simulink model "hil_vhf_model_setup"  (R2022b)
settings: Solver=FixedStepAuto  StartTime=0.0  StopTime=9  RelTol=1e-3
PreLoadFcn:
  | run('control_bus.m')
  | addpath('.\observers','.\control')
model workspace (MAT data in the model file):
  C = 39.8
  D = 0.05
  Lc = [1.1848250893; -624.760865246]
  M = 740
  Nd = 40
  Tmax = 1000
  a = 0.015
  esc_ic = 0.1
  g = 9.807
  h = 0.577
  l = 1.917
  lf = 1.036
  lr = 0.881
  omega = 100
  phi = -1.0471975512
  re = 0.284
  x0 = 200
  x_c = 90
  x_l = 10
undefined symbols (not defined in the file): Kalman, magnitude, r
libraries: simulink x2, Solver_SF x1
CloseFcn:
  | clear control_info_bus
settings Model: DataDictionary=kf_dict.sldd  Creator=henri  LastModifiedBy=Henrique Mesquita
settings DebuggingCC: UnconnectedInputMsg=warning  UnconnectedOutputMsg=warning  UnconnectedLineMsg=warning
settings ModelReferenceCC: EnableRefExpFcnMdlSchedulingChecks=on
settings SFSimCC: SimUserIncludeDirs="\".\\observers\""
settings RTWCC: DLArmComputeVersion=19.05

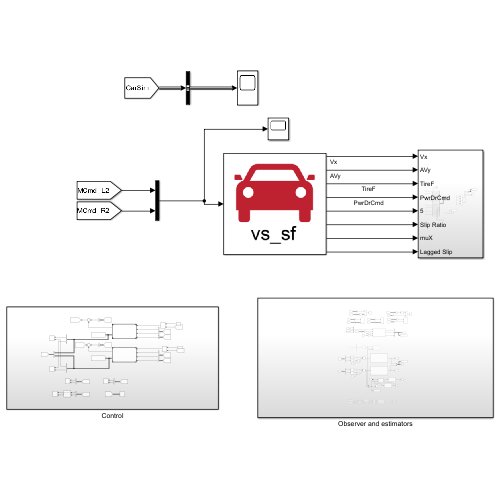
[thumbnail: Simulink's stored preview of the top-level diagram]
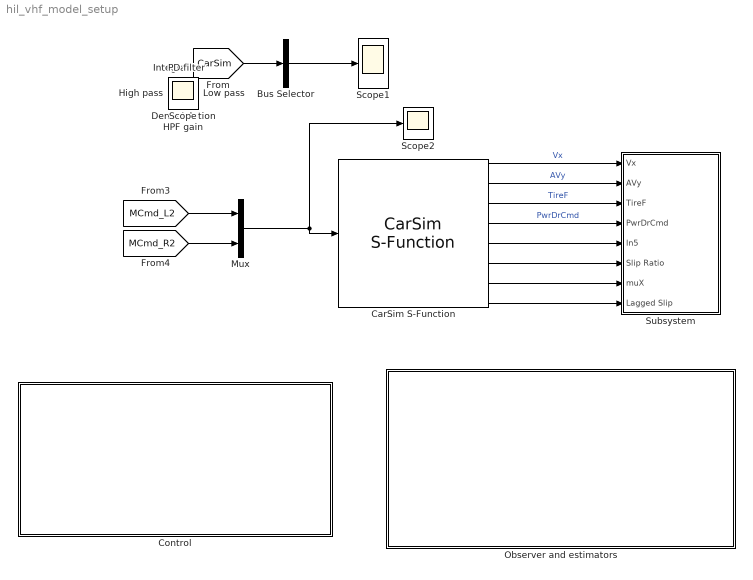
== system hil_vhf_model_setup ==
  Bus Selector : BusSelector  OutputSignals=AVy_L1,AVy_R1,AVy_L2,AVy_R2  OutputAsBus=on
  CarSim S-Function : Solver_SF/CarSim S-Function  Priority=1  SIMFILE=simfile.sim  Run_RTs=off  vs_state_ind=Run  StopMode_ind=Vehicle Model
  Control : Subsystem
  Mux : Mux  Inputs=2
  Observer and estimators : Subsystem
  Scope1 : Scope
  Scope2 : Scope
  Subsystem : Subsystem
  Demodulation : Scope
  HPF gain : Scope
  High pass : Scope
  Integrator : Scope
  Low pass : Scope
  PD filter : Scope
  Scope : Scope
  wires:
  Mux/1 -> Scope2/1, CarSim S-Function/1
  [CarSim] -> Bus Selector/1
  Bus Selector/1 -> Scope1/1
  CarSim S-Function/2 -> Subsystem/2(AVy)  "AVy"
  [MCmd_R2] -> Mux/2
  [MCmd_L2] -> Mux/1
  CarSim S-Function/6 -> Subsystem/6(Slip Ratio)
  CarSim S-Function/7 -> Subsystem/7(muX)
  CarSim S-Function/1 -> Subsystem/1(Vx)  "Vx"
  CarSim S-Function/3 -> Subsystem/3(TireF)  "TireF"
  CarSim S-Function/4 -> Subsystem/4(PwrDrCmd)  "PwrDrCmd"
  CarSim S-Function/5 -> Subsystem/5(In5)
  CarSim S-Function/8 -> Subsystem/8(Lagged Slip)

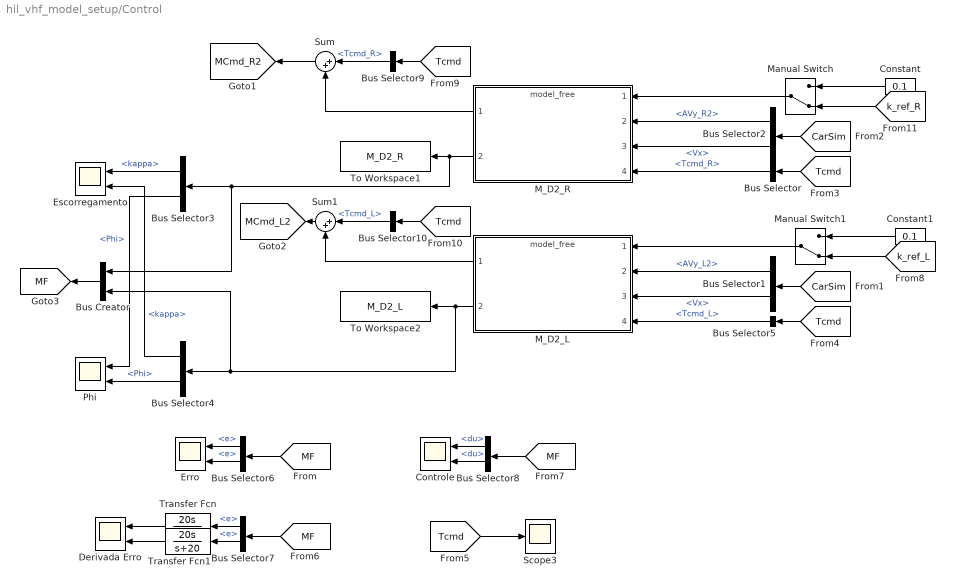
== system hil_vhf_model_setup/Control ==
  Bus Creator : BusCreator  Inputs=2
  Bus Selector : BusSelector  OutputSignals=Tcmd_R
  Bus Selector1 : BusSelector  OutputSignals=AVy_L2,Vx
  Bus Selector10 : BusSelector  OutputSignals=Tcmd_L
  Bus Selector2 : BusSelector  OutputSignals=AVy_R2,Vx
  Bus Selector3 : BusSelector  OutputSignals=kappa,Phi
  Bus Selector4 : BusSelector  OutputSignals=kappa,Phi
  Bus Selector5 : BusSelector  OutputSignals=Tcmd_L
  Bus Selector6 : BusSelector  OutputSignals=info (signal 1).e,info (signal 2).e
  Bus Selector7 : BusSelector  OutputSignals=info (signal 1).e,info (signal 2).e
  Bus Selector8 : BusSelector  OutputSignals=info (signal 1).du,info (signal 2).du
  Bus Selector9 : BusSelector  OutputSignals=Tcmd_R
  Constant : Constant  Value=0.1
  Constant1 : Constant  Value=0.1
  Controle : Scope  NumInputPorts=2
  Derivada Erro : Scope  NumInputPorts=2
  Erro : Scope  NumInputPorts=2
  "Escorregamento " : Scope  NumInputPorts=2
  M_D2_L : ModelReference  ModelNameDialog=model_free.slx  SimulationMode=Normal  ModelReferenceVersion=4.1
  M_D2_R : ModelReference  ModelNameDialog=model_free.slx  SimulationMode=Normal  ModelReferenceVersion=4.1
  Manual Switch : ManualSwitch  CurrentSetting=0
  Manual Switch1 : ManualSwitch  CurrentSetting=0
  Phi : Scope  NumInputPorts=2
  Scope3 : Scope
  Sum : Sum  Inputs=|++
  Sum1 : Sum  Inputs=|++
  To Workspace1 : ToWorkspace  VariableName=M_D2_R  SaveFormat=Timeseries  SampleTime=-1
  To Workspace2 : ToWorkspace  VariableName=M_D2_L  SaveFormat=Timeseries  SampleTime=-1
  Transfer Fcn : TransferFcn  Numerator=[20 0]  Denominator=[1 20]
  Transfer Fcn1 : TransferFcn  Numerator=[20 0]  Denominator=[1 20]
  tag scope: MCmd_L2=global, MCmd_R2=global, MF=global
  wires:
  M_D2_R/2 -> Bus Creator/1, Bus Selector3/1, To Workspace1/1
  Bus Selector3/1 -> "Escorregamento "/1  "<kappa>"
  Bus Selector1/1 -> M_D2_L/2  "<AVy_L2>"
  M_D2_L/2 -> Bus Creator/2, Bus Selector4/1, To Workspace2/1
  Manual Switch/1 -> M_D2_R/1
  Bus Selector4/2 -> Phi/2  "<Phi>"
  Bus Selector4/1 -> "Escorregamento "/2  "<kappa>"
  [CarSim] -> Bus Selector1/1
  Bus Selector3/2 -> Phi/1  "<Phi>"
  Bus Selector1/2 -> M_D2_L/3  "<Vx>"
  [CarSim] -> Bus Selector2/1
  Bus Selector2/1 -> M_D2_R/2  "<AVy_R2>"
  Bus Selector2/2 -> M_D2_R/3  "<Vx>"
  [Tcmd] -> Bus Selector/1
  Bus Selector/1 -> M_D2_R/4  "<Tcmd_R>"
  [Tcmd] -> Bus Selector5/1
  Bus Selector5/1 -> M_D2_L/4  "<Tcmd_L>"
  [Tcmd] -> Scope3/1
  [k_ref_R] -> Manual Switch/2
  Constant/1 -> Manual Switch/1
  Bus Creator/1 -> [MF]
  [MF] -> Bus Selector6/1
  Bus Selector6/1 -> Erro/1  "<e>"
  Bus Selector6/2 -> Erro/2  "<e>"
  [MF] -> Bus Selector7/1
  Bus Selector7/2 -> Transfer Fcn1/1  "<e>"
  Bus Selector7/1 -> Transfer Fcn/1  "<e>"
  Transfer Fcn/1 -> Derivada Erro/1
  Transfer Fcn1/1 -> Derivada Erro/2
  Bus Selector8/2 -> Controle/2  "<du>"
  Bus Selector8/1 -> Controle/1  "<du>"
  [MF] -> Bus Selector8/1
  Constant1/1 -> Manual Switch1/1
  [k_ref_L] -> Manual Switch1/2
  Manual Switch1/1 -> M_D2_L/1
  Sum/1 -> [MCmd_R2]
  [Tcmd] -> Bus Selector9/1
  Bus Selector9/1 -> Sum/1  "<Tcmd_R>"
  M_D2_R/1 -> Sum/2
  Bus Selector10/1 -> Sum1/1  "<Tcmd_L>"
  [Tcmd] -> Bus Selector10/1
  Sum1/1 -> [MCmd_L2]
  M_D2_L/1 -> Sum1/2

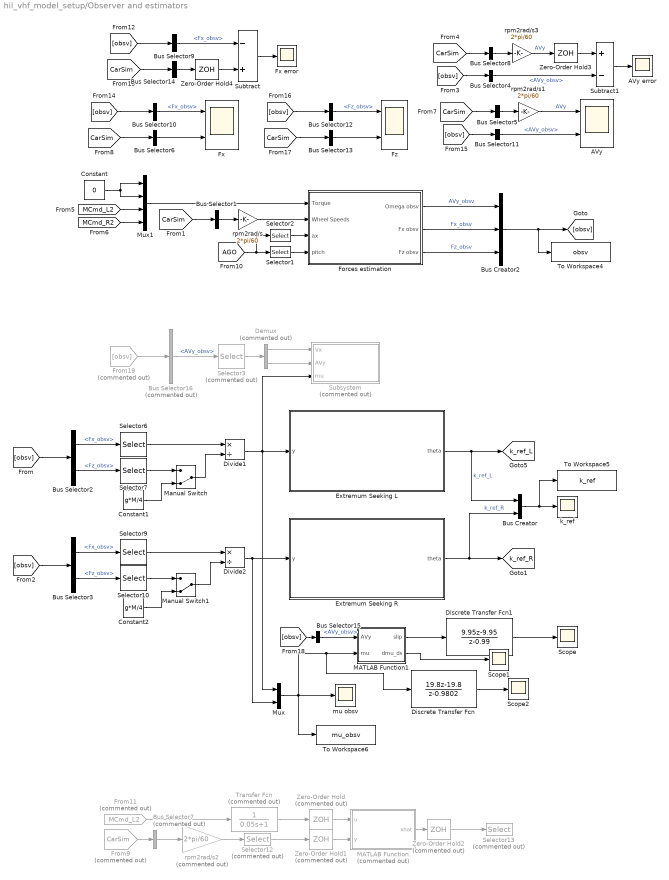
== system hil_vhf_model_setup/Observer and estimators ==
  AVy : Scope  NumInputPorts=2
  AVy error : Scope
  Bus Creator : BusCreator  Inputs=2
  Bus Creator2 : BusCreator  Inputs=3
  Bus Selector1 : BusSelector  OutputSignals=AVy_L1,AVy_R1,AVy_L2,AVy_R2  OutputAsBus=on
  Bus Selector10 : BusSelector  OutputSignals=Fx_obsv
  Bus Selector11 : BusSelector  OutputSignals=AVy_obsv
  Bus Selector12 : BusSelector  OutputSignals=Fz_obsv
  Bus Selector13 : BusSelector  OutputSignals=Fz_L1,Fz_R1,Fz_L2,Fz_R2  OutputAsBus=on
  Bus Selector14 : BusSelector  OutputSignals=Fx_L1,Fx_R1,Fx_L2,Fx_R2  OutputAsBus=on
  Bus Selector15 : BusSelector  OutputSignals=AVy_obsv
  Bus Selector16 : BusSelector  Commented=on  OutputSignals=AVy_obsv
  Bus Selector2 : BusSelector  OutputSignals=Fx_obsv,Fz_obsv
  Bus Selector3 : BusSelector  OutputSignals=Fx_obsv,Fz_obsv
  Bus Selector4 : BusSelector  OutputSignals=AVy_obsv
  Bus Selector5 : BusSelector  OutputSignals=AVy_L1,AVy_R1,AVy_L2,AVy_R2  OutputAsBus=on
  Bus Selector6 : BusSelector  OutputSignals=Fx_L1,Fx_R1,Fx_L2,Fx_R2  OutputAsBus=on
  Bus Selector7 : BusSelector  Commented=on  OutputSignals=AVy_L1,AVy_R1,AVy_L2,AVy_R2  OutputAsBus=on
  Bus Selector8 : BusSelector  OutputSignals=AVy_L1,AVy_R1,AVy_L2,AVy_R2  OutputAsBus=on
  Bus Selector9 : BusSelector  OutputSignals=Fx_obsv
  Constant : Constant  Value=0
  Constant1 : Constant  Value=g*M/4
  Constant2 : Constant  Value=g*M/4
  Demux : Demux  Commented=on  Outputs=2
  Discrete Transfer Fcn : DiscreteTransferFcn  Numerator=[19.8 -19.8]  Denominator=[1 -0.9802]
  Discrete Transfer Fcn1 : DiscreteTransferFcn  Numerator=[9.95 -9.95]  Denominator=[1 -0.99]
  Divide1 : Product  Inputs=*/
  Divide2 : Product  Inputs=*/
  Extremum Seeking L : Subsystem  Variant=on  VariantControlMode=label  VariantControl=Choice  LabelModeActiveChoice=ESC w/ vx gain  PropagateVariantConditions=on
  Extremum Seeking R : Subsystem  Variant=on  VariantControlMode=label  VariantControl=Choice  LabelModeActiveChoice=ESC w/ vx gain  PropagateVariantConditions=on
  Forces estimation : Subsystem  Variant=on  VariantControlMode=label  VariantControl=Choice  LabelModeActiveChoice=algebraic_PIO
  From11 : From  Commented=on  GotoTag=MCmd_L2  TagVisibility=global
  From19 : From  Commented=on  GotoTag=obsv
  From9 : From  Commented=on  GotoTag=CarSim  TagVisibility=global
  Fx : Scope  NumInputPorts=2
  Fx error : Scope
  Fz : Scope  NumInputPorts=2
  MATLAB Function : MATLAB Function  Commented=on  TreatAsAtomicUnit=on
  MATLAB Function1 : MATLAB Function  TreatAsAtomicUnit=on
  Manual Switch : ManualSwitch  CurrentSetting=0
  Manual Switch1 : ManualSwitch  CurrentSetting=0
  Mux : Mux  Inputs=2
  Mux1 : Mux
  Scope : Scope
  Scope1 : Scope
  Scope2 : Scope
  Selector1 : Selector  InputPortWidth=9  IndexOptions=Index vector (dialog)  Indices=[8]  OutputSizes=1
  Selector10 : Selector  InputPortWidth=4  IndexOptions=Index vector (dialog)  Indices=[4]  OutputSizes=1
  Selector12 : Selector  Commented=on  InputPortWidth=4  IndexOptions=Index vector (dialog)  Indices=[3]  OutputSizes=1
  Selector13 : Selector  Commented=on  InputPortWidth=2  IndexOptions=Index vector (dialog)  Indices=[2]  OutputSizes=1
  Selector2 : Selector  InputPortWidth=9  IndexOptions=Index vector (dialog)  Indices=[1]  OutputSizes=1
  Selector3 : Selector  Commented=on  InputPortWidth=4  IndexOptions=Index vector (dialog)  Indices=[1 3]  OutputSizes=1
  Selector6 : Selector  InputPortWidth=4  IndexOptions=Index vector (dialog)  Indices=[3]  OutputSizes=1
  Selector7 : Selector  InputPortWidth=4  IndexOptions=Index vector (dialog)  Indices=[3]  OutputSizes=1
  Selector9 : Selector  InputPortWidth=4  IndexOptions=Index vector (dialog)  Indices=[4]  OutputSizes=1
  Subsystem : Subsystem  Commented=on
  Subtract : Sum  Inputs=-+
  Subtract1 : Sum  Inputs=+-
  To Workspace4 : ToWorkspace  VariableName=obsv  SaveFormat=Timeseries  SampleTime=-1
  To Workspace5 : ToWorkspace  VariableName=k_ref  SaveFormat=Timeseries  SampleTime=-1
  To Workspace6 : ToWorkspace  VariableName=mu_obsv  SaveFormat=Timeseries  SampleTime=-1
  Transfer Fcn : TransferFcn  Commented=on  Denominator=[0.05 1]
  Zero-Order Hold : ZeroOrderHold  Commented=on  SampleTime=0.001
  Zero-Order Hold1 : ZeroOrderHold  Commented=on  SampleTime=0.001
  Zero-Order Hold2 : ZeroOrderHold  Commented=on  SampleTime=0.001
  Zero-Order Hold3 : ZeroOrderHold  SampleTime=0.001
  Zero-Order Hold4 : ZeroOrderHold  SampleTime=0.001
  k_ref : Scope
  mu obsv : Scope
  rpm2rad/s : Gain  Gain=2*pi/60
  rpm2rad/s1 : Gain  Gain=2*pi/60
  rpm2rad/s2 : Gain  Commented=on  Gain=2*pi/60
  rpm2rad/s3 : Gain  Gain=2*pi/60
  tag scope: k_ref_L=global, k_ref_R=global
  wires:
  Bus Creator2/1 -> To Workspace4/1, [obsv]
  Bus Selector5/1 -> rpm2rad/s1/1
  Bus Selector1/1 -> rpm2rad/s/1
  [MCmd_R2] -> Mux1/4
  [CarSim] -> Bus Selector5/1
  [CarSim] -> Bus Selector6/1
  [AGO] -> Selector2/1, Selector1/1
  Bus Selector6/1 -> Fx/2
  [MCmd_L2] -> Mux1/3
  [CarSim] -> Bus Selector1/1
  Constant/1 -> Mux1/2, Mux1/1
  rpm2rad/s1/1 -> AVy/1  "AVy"
  Extremum Seeking L/1(theta) -> Bus Creator/1, [k_ref_L]  "k_ref_L"
  From9/1 -> Bus Selector7/1
  Bus Selector7/1 -> rpm2rad/s2/1
  rpm2rad/s2/1 -> Selector12/1
  Zero-Order Hold1/1 -> MATLAB Function/2(y)
  MATLAB Function/1(xhat) -> Zero-Order Hold2/1
  [obsv] -> Bus Selector10/1
  Bus Selector10/1 -> Fx/1  "<Fx_obsv>"
  [obsv] -> Bus Selector11/1
  Bus Selector11/1 -> AVy/2  "<AVy_obsv>"
  From11/1 -> Transfer Fcn/1
  Selector12/1 -> Zero-Order Hold1/1
  Zero-Order Hold2/1 -> Selector13/1
  Zero-Order Hold/1 -> MATLAB Function/1(u)
  [obsv] -> Bus Selector12/1
  Bus Selector13/1 -> Fz/2
  [CarSim] -> Bus Selector13/1
  Bus Selector12/1 -> Fz/1  "<Fz_obsv>"
  Transfer Fcn/1 -> Zero-Order Hold/1
  Extremum Seeking R/1(theta) -> Bus Creator/2, [k_ref_R]  "k_ref_R"
  Bus Creator/1 -> To Workspace5/1, k_ref/1
  Mux1/1 -> Forces estimation/1(Torque)
  rpm2rad/s/1 -> Forces estimation/2(Wheel Speeds)
  Selector2/1 -> Forces estimation/3(ax)
  Selector1/1 -> Forces estimation/4(pitch)
  Forces estimation/1(Omega obsv) -> Bus Creator2/1  "AVy_obsv"
  Forces estimation/2(Fx obsv) -> Bus Creator2/2  "Fx_obsv"
  Forces estimation/3(Fz obsv) -> Bus Creator2/3  "Fz_obsv"
  [obsv] -> Bus Selector2/1
  Bus Selector2/1 -> Selector6/1  "<Fx_obsv>"
  Bus Selector2/2 -> Selector7/1  "<Fz_obsv>"
  Selector6/1 -> Divide1/1
  Divide1/1 -> Subsystem/3(mu), Mux/1, Extremum Seeking L/1(y)
  Bus Selector3/1 -> Selector9/1  "<Fx_obsv>"
  [obsv] -> Bus Selector3/1
  Selector9/1 -> Divide2/1
  Bus Selector3/2 -> Selector10/1  "<Fz_obsv>"
  Divide2/1 -> Mux/2, Extremum Seeking R/1(y)
  Mux/1 -> Discrete Transfer Fcn/1, MATLAB Function1/2(mu), To Workspace6/1, mu obsv/1
  Manual Switch/1 -> Divide1/2
  Selector7/1 -> Manual Switch/1
  Constant1/1 -> Manual Switch/2
  Constant2/1 -> Manual Switch1/2
  Manual Switch1/1 -> Divide2/2
  Selector10/1 -> Manual Switch1/1
  Subtract/1 -> Fx error/1
  Subtract1/1 -> AVy error/1
  [CarSim] -> Bus Selector8/1
  Bus Selector8/1 -> rpm2rad/s3/1
  [obsv] -> Bus Selector4/1
  Bus Selector4/1 -> Subtract1/2  "<AVy_obsv>"
  rpm2rad/s3/1 -> Zero-Order Hold3/1  "AVy"
  Zero-Order Hold3/1 -> Subtract1/1
  [obsv] -> Bus Selector9/1
  [CarSim] -> Bus Selector14/1
  Bus Selector14/1 -> Zero-Order Hold4/1
  Zero-Order Hold4/1 -> Subtract/2
  Bus Selector9/1 -> Subtract/1  "<Fx_obsv>"
  [obsv] -> Bus Selector15/1
  Bus Selector15/1 -> MATLAB Function1/1(AVy)  "<AVy_obsv>"
  MATLAB Function1/1(slip) -> Discrete Transfer Fcn1/1
  MATLAB Function1/2(dmu_ds) -> Scope1/1
  Discrete Transfer Fcn/1 -> Scope2/1
  Discrete Transfer Fcn1/1 -> Scope/1
  From19/1 -> Bus Selector16/1
  Bus Selector16/1 -> Selector3/1  "<AVy_obsv>"
  Selector3/1 -> Demux/1
  Demux/1 -> Subsystem/1(Vx)
  Demux/2 -> Subsystem/2(AVy)

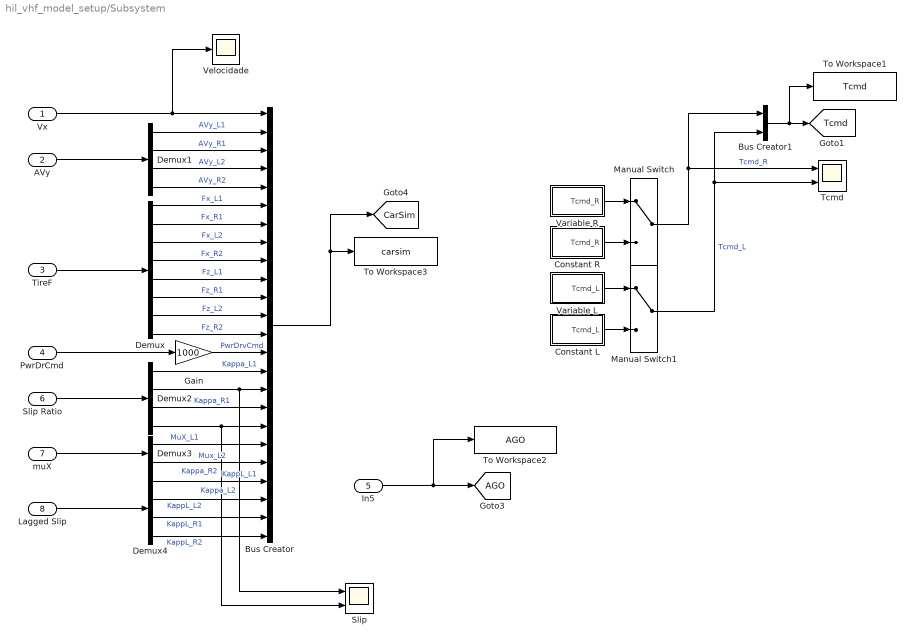
== system hil_vhf_model_setup/Subsystem ==
  Vx : Inport
  AVy : Inport  Port=2
  TireF : Inport  Port=3
  PwrDrCmd : Inport  Port=4
  In5 : Inport  Port=5
  Slip Ratio : Inport  Port=6
  muX : Inport  Port=7
  Lagged Slip : Inport  Port=8
  Bus Creator : BusCreator  Inputs=24
  Bus Creator1 : BusCreator  Inputs=2
  Constant L : Subsystem
  Constant R : Subsystem
  Demux : Demux  Outputs=8
  Demux1 : Demux
  Demux2 : Demux
  Demux3 : Demux  Outputs=2
  Demux4 : Demux
  Gain : Gain  Gain=1000
  Manual Switch : ManualSwitch
  Manual Switch1 : ManualSwitch
  Slip : Scope  NumInputPorts=2
  Tcmd : Scope  NumInputPorts=2
  To Workspace1 : ToWorkspace  VariableName=Tcmd  SaveFormat=Timeseries  SampleTime=-1
  To Workspace2 : ToWorkspace  VariableName=AGO  SaveFormat=Timeseries  SampleTime=-1
  To Workspace3 : ToWorkspace  VariableName=carsim  SaveFormat=Timeseries  SampleTime=-1
  Variable L : Subsystem
  Variable R : Subsystem
  Velocidade : Scope
  tag scope: AGO=global, CarSim=global, Tcmd=global
  wires:
  In5/1 -> To Workspace2/1, [AGO]
  Bus Creator/1 -> [CarSim], To Workspace3/1
  Demux2/4 -> Bus Creator/18, Slip/2  "Kappa_R2"
  Demux2/3 -> Bus Creator/17  "Kappa_R1"
  Slip Ratio/1 -> Demux2/1
  AVy/1 -> Demux1/1
  Demux2/2 -> Bus Creator/16, Slip/1  "Kappa_L2"
  Demux2/1 -> Bus Creator/15  "Kappa_L1"
  Demux/2 -> Bus Creator/7  "Fx_R1"
  PwrDrCmd/1 -> Gain/1
  Demux1/1 -> Bus Creator/2  "AVy_L1"
  Demux1/2 -> Bus Creator/3  "AVy_R1"
  Demux/1 -> Bus Creator/6  "Fx_L1"
  Demux1/3 -> Bus Creator/4  "AVy_L2"
  TireF/1 -> Demux/1
  Demux1/4 -> Bus Creator/5  "AVy_R2"
  Vx/1 -> Velocidade/1, Bus Creator/1
  Gain/1 -> Bus Creator/14  "PwrDrvCmd"
  Demux/3 -> Bus Creator/8  "Fx_L2"
  Demux/4 -> Bus Creator/9  "Fx_R2"
  Demux3/1 -> Bus Creator/19  "MuX_L1"
  Demux3/2 -> Bus Creator/20  "Mux_L2"
  muX/1 -> Demux3/1
  Demux/5 -> Bus Creator/10  "Fz_L1"
  Demux/6 -> Bus Creator/11  "Fz_R1"
  Demux/7 -> Bus Creator/12  "Fz_L2"
  Demux/8 -> Bus Creator/13  "Fz_R2"
  Constant L/1(Tcmd_L) -> Manual Switch1/2
  Variable L/1(Tcmd_L) -> Manual Switch1/1
  Manual Switch1/1 -> Bus Creator1/2, Tcmd/2  "Tcmd_L"
  Constant R/1(Tcmd_R) -> Manual Switch/2
  Bus Creator1/1 -> To Workspace1/1, [Tcmd]
  Variable R/1(Tcmd_R) -> Manual Switch/1
  Manual Switch/1 -> Bus Creator1/1, Tcmd/1  "Tcmd_R"
  Lagged Slip/1 -> Demux4/1
  Demux4/1 -> Bus Creator/21  "KappL_L1"
  Demux4/2 -> Bus Creator/22  "KappL_L2"
  Demux4/3 -> Bus Creator/23  "KappL_R1"
  Demux4/4 -> Bus Creator/24  "KappL_R2"

== system hil_vhf_model_setup/Observer and estimators/Extremum Seeking L ==
  y : Inport
  ESC w/ derivative : Subsystem  VariantControl=Choice 2
  Extremum Seeking vx gain : Subsystem  VariantControl=ESC w/ vx gain  ReferencedSubsystem=Extremum_Seeking_vx_gain
      settings: MinAlgLoopOccurrences=on
  Perturbation ESC : Subsystem  VariantControl=Choice 1  ReferencedSubsystem=Perturbation_ESC
  Slope Seeking : Subsystem  VariantControl=Choice 3
  theta : Outport

== system hil_vhf_model_setup/Observer and estimators/Extremum Seeking R ==
  y : Inport
  ESC w/ derivative : Subsystem  VariantControl=Choice 2
  Extremum Seeking vx gain : Subsystem  VariantControl=ESC w/ vx gain  ReferencedSubsystem=Extremum_Seeking_vx_gain
      settings: MinAlgLoopOccurrences=on
  Perturbation ESC : Subsystem  VariantControl=Choice 1  ReferencedSubsystem=Perturbation_ESC
  Slope Seeking : Subsystem  VariantControl=Choice 3
  theta : Outport

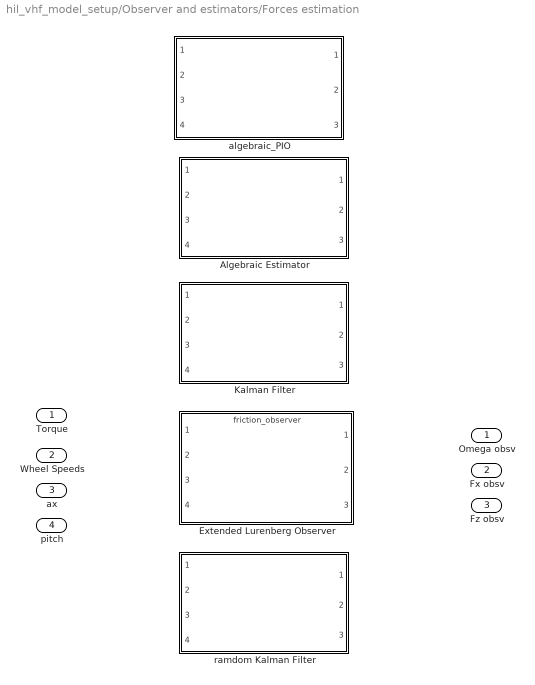
== system hil_vhf_model_setup/Observer and estimators/Forces estimation ==
  Torque : Inport
  Wheel Speeds : Inport  Port=2
  ax : Inport  Port=3
  pitch : Inport  Port=4
  Algebraic Estimator : Subsystem  TreatAsAtomicUnit=on  VariantControl=Alg_Est  ReferencedSubsystem=Force_algebraic_estimator
  Extended Lurenberg Observer : ModelReference  ModelNameDialog=friction_observer.slx  SimulationMode=Normal  VariantControl=Ext Lurenberg  ModelReferenceVersion=1.10
  Kalman Filter : Subsystem  TreatAsAtomicUnit=on  VariantControl=Kalman  ReferencedSubsystem=Kalman_Filter
  algebraic_PIO : Subsystem  TreatAsAtomicUnit=on  VariantControl=algebraic_PIO  ReferencedSubsystem=algebraic_PIO_observer
  ramdom Kalman Filter : Subsystem  TreatAsAtomicUnit=on  VariantControl=r-Kalman  ReferencedSubsystem=r_Kalman_Filter
  Omega obsv : Outport
  Fx obsv : Outport  Port=2
  Fz obsv : Outport  Port=3

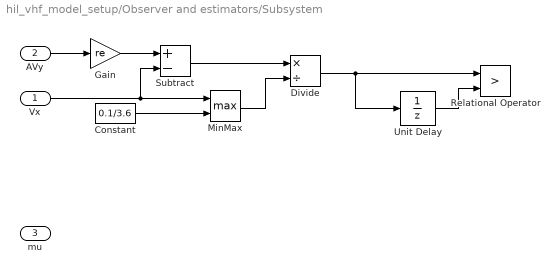
== system hil_vhf_model_setup/Observer and estimators/Subsystem ==
  Vx : Inport
  AVy : Inport  Port=2
  mu : Inport  Port=3
  Constant : Constant  Value=0.1/3.6
  Divide : Product  Inputs=*/
  Gain : Gain  Gain=re
  MinMax : MinMax  Function=max  Inputs=2
  Relational Operator : RelationalOperator  Operator=>  OutDataTypeStr=boolean  RndMeth=Simplest  InputSameDT=off
  Subtract : Sum  Inputs=+-
  Unit Delay : UnitDelay  SampleTime=0.001  HasFrameUpgradeWarning=on
  wires:
  AVy/1 -> Gain/1
  Gain/1 -> Subtract/1
  Vx/1 -> MinMax/1, Subtract/2
  Constant/1 -> MinMax/2
  Subtract/1 -> Divide/1
  MinMax/1 -> Divide/2
  Divide/1 -> Relational Operator/1, Unit Delay/1
  Unit Delay/1 -> Relational Operator/2

== system hil_vhf_model_setup/Subsystem/Constant L ==
  Bus Selector1 : BusSelector  OutputSignals=PwrDrvCmd
  Gain1 : Gain  Gain=1/20000
  Gain2 : Gain  Gain=Tmax
  Tcmd_L : Outport
  wires:
  Gain2/1 -> Tcmd_L/1  "Tcmd_L"
  Gain1/1 -> Gain2/1  "throttle"
  [CarSim] -> Bus Selector1/1
  Bus Selector1/1 -> Gain1/1  "<PwrDrvCmd>"

== system hil_vhf_model_setup/Subsystem/Constant R ==
  Bus Selector1 : BusSelector  OutputSignals=PwrDrvCmd
  Gain1 : Gain  Gain=1/20000
  Gain2 : Gain  Gain=Tmax
  Tcmd_R : Outport
  wires:
  Gain2/1 -> Tcmd_R/1  "Tcmd_R"
  Gain1/1 -> Gain2/1  "throttle"
  [CarSim] -> Bus Selector1/1
  Bus Selector1/1 -> Gain1/1  "<PwrDrvCmd>"

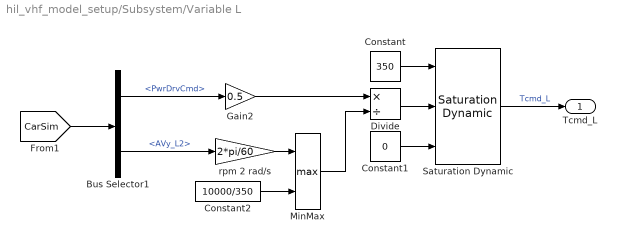
== system hil_vhf_model_setup/Subsystem/Variable L ==
  Bus Selector1 : BusSelector  OutputSignals=PwrDrvCmd,AVy_L2
  Constant : Constant  Value=350
  Constant1 : Constant  Value=0
  Constant2 : Constant  Value=10000/350
  Divide : Product  Inputs=*/
  Gain2 : Gain  Gain=0.5
  MinMax : MinMax  Function=max  Inputs=2
  Saturation Dynamic : simulink/Discontinuities/Saturation Dynamic  OutMin=[]  OutMax=[]  OutDataTypeStr=Inherit: Same as second input  OutDataType=fixdt(1, 16)  OutScaling=2^-10  DoSatur=off
  rpm 2 rad/s : Gain  Gain=2*pi/60
  Tcmd_L : Outport
  wires:
  [CarSim] -> Bus Selector1/1
  Bus Selector1/1 -> Gain2/1  "<PwrDrvCmd>"
  Divide/1 -> Saturation Dynamic/2
  Constant1/1 -> Saturation Dynamic/3
  Bus Selector1/2 -> rpm 2 rad/s/1  "<AVy_L2>"
  Gain2/1 -> Divide/1
  Saturation Dynamic/1 -> Tcmd_L/1  "Tcmd_L"
  rpm 2 rad/s/1 -> MinMax/1
  MinMax/1 -> Divide/2
  Constant2/1 -> MinMax/2
  Constant/1 -> Saturation Dynamic/1

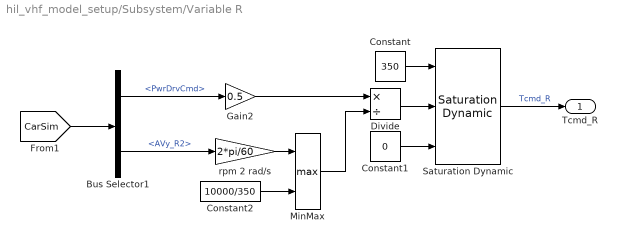
== system hil_vhf_model_setup/Subsystem/Variable R ==
  Bus Selector1 : BusSelector  OutputSignals=PwrDrvCmd,AVy_R2
  Constant : Constant  Value=350
  Constant1 : Constant  Value=0
  Constant2 : Constant  Value=10000/350
  Divide : Product  Inputs=*/
  Gain2 : Gain  Gain=0.5
  MinMax : MinMax  Function=max  Inputs=2
  Saturation Dynamic : simulink/Discontinuities/Saturation Dynamic  OutMin=[]  OutMax=[]  OutDataTypeStr=Inherit: Same as second input  OutDataType=fixdt(1, 16)  OutScaling=2^-10  DoSatur=off
  rpm 2 rad/s : Gain  Gain=2*pi/60
  Tcmd_R : Outport
  wires:
  [CarSim] -> Bus Selector1/1
  Bus Selector1/1 -> Gain2/1  "<PwrDrvCmd>"
  Divide/1 -> Saturation Dynamic/2
  Constant1/1 -> Saturation Dynamic/3
  Bus Selector1/2 -> rpm 2 rad/s/1  "<AVy_R2>"
  Constant/1 -> Saturation Dynamic/1
  Gain2/1 -> Divide/1
  Saturation Dynamic/1 -> Tcmd_R/1  "Tcmd_R"
  rpm 2 rad/s/1 -> MinMax/1
  MinMax/1 -> Divide/2
  Constant2/1 -> MinMax/2

== system hil_vhf_model_setup/Observer and estimators/Extremum Seeking L/ESC w// derivative ==
  y : Inport
  Extremum Seeking : Subsystem
  Gain : Gain  Gain=1/(g*M/4)
  Math Function : Math  Commented=through  Operator=magnitude^2
  Transfer Fcn : TransferFcn  Commented=through  Numerator=[80]  Denominator=[1 80]
  theta : Outport
  wires:
  Transfer Fcn/1 -> Gain/1
  Gain/1 -> Math Function/1  "mu_obsv"
  Extremum Seeking/1(theta) -> theta/1
  Math Function/1 -> Extremum Seeking/1(y)  "mu_obsv"
  y/1 -> Transfer Fcn/1

== system hil_vhf_model_setup/Observer and estimators/Extremum Seeking L/Slope Seeking ==
  y : Inport
  Gain : Gain  Gain=1/(g*M/4)
  Math Function : Math  Operator=magnitude^2
  Slope Seeking : Subsystem
  Transfer Fcn : TransferFcn  Commented=through  Numerator=[80]  Denominator=[1 80]
  theta : Outport
  wires:
  Transfer Fcn/1 -> Gain/1
  Gain/1 -> Math Function/1  "mu_obsv"
  Slope Seeking/1(theta) -> theta/1
  Math Function/1 -> Slope Seeking/1(y)  "mu_obsv"
  y/1 -> Transfer Fcn/1

== system hil_vhf_model_setup/Observer and estimators/Extremum Seeking R/ESC w// derivative ==
  y : Inport
  Extremum Seeking : Subsystem
  Gain : Gain  Gain=1/(g*M/4)
  Math Function : Math  Commented=through  Operator=magnitude^2
  Transfer Fcn : TransferFcn  Commented=through  Numerator=[80]  Denominator=[1 80]
  theta : Outport
  wires:
  Transfer Fcn/1 -> Gain/1
  Gain/1 -> Math Function/1  "mu_obsv"
  Extremum Seeking/1(theta) -> theta/1
  Math Function/1 -> Extremum Seeking/1(y)  "mu_obsv"
  y/1 -> Transfer Fcn/1

== system hil_vhf_model_setup/Observer and estimators/Extremum Seeking R/Slope Seeking ==
  y : Inport
  Gain : Gain  Gain=1/(g*M/4)
  Math Function : Math  Operator=magnitude^2
  Slope Seeking : Subsystem
  Transfer Fcn : TransferFcn  Commented=through  Numerator=[80]  Denominator=[1 80]
  theta : Outport
  wires:
  Transfer Fcn/1 -> Gain/1
  Gain/1 -> Math Function/1  "mu_obsv"
  Slope Seeking/1(theta) -> theta/1
  Math Function/1 -> Slope Seeking/1(y)  "mu_obsv"
  y/1 -> Transfer Fcn/1

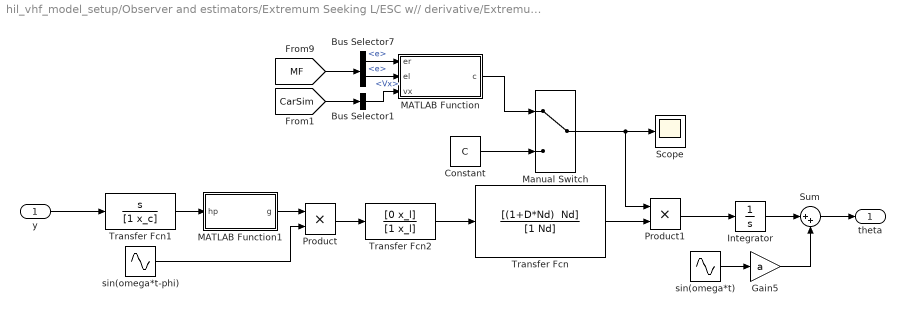
== system hil_vhf_model_setup/Observer and estimators/Extremum Seeking L/ESC w// derivative/Extremum Seeking ==
  y : Inport
  Bus Selector1 : BusSelector  OutputSignals=Vx
  Bus Selector7 : BusSelector  OutputSignals=info (signal 1).e,info (signal 2).e
  Constant : Constant  Value=C
  Gain5 : Gain  Gain=a
  Integrator : Integrator  InitialCondition=0.1  LimitOutput=on  UpperSaturationLimit=0.1  LowerSaturationLimit=0.099
  MATLAB Function : MATLAB Function  TreatAsAtomicUnit=on
  MATLAB Function1 : MATLAB Function  TreatAsAtomicUnit=on
  Manual Switch : ManualSwitch
  Product : Product
  Product1 : Product
  Scope : Scope
  Sum : Sum  Inputs=|++
  Transfer Fcn : TransferFcn  Numerator="[(1+D*Nd)  Nd]"  Denominator=[1 Nd]
  Transfer Fcn1 : TransferFcn  Numerator=[1 0]  Denominator=[1 x_c]
  Transfer Fcn2 : TransferFcn  Numerator=[0 x_l]  Denominator=[1 x_l]
  sin(omega*t) : Sin  Frequency=omega  SampleTime=0
  sin(omega*t-phi) : Sin  Frequency=omega  Phase=phi  SampleTime=0
  theta : Outport
  wires:
  sin(omega*t)/1 -> Gain5/1
  Gain5/1 -> Sum/2
  Sum/1 -> theta/1
  Product/1 -> Transfer Fcn2/1
  y/1 -> Transfer Fcn1/1
  sin(omega*t-phi)/1 -> Product/2
  Product1/1 -> Integrator/1
  Integrator/1 -> Sum/1
  [MF] -> Bus Selector7/1
  Bus Selector7/1 -> MATLAB Function/1(er)  "<e>"
  Bus Selector7/2 -> MATLAB Function/2(el)  "<e>"
  MATLAB Function/1(c) -> Manual Switch/1
  Constant/1 -> Manual Switch/2
  Manual Switch/1 -> Product1/1, Scope/1
  Transfer Fcn1/1 -> MATLAB Function1/1(hp)
  [CarSim] -> Bus Selector1/1
  Bus Selector1/1 -> MATLAB Function/3(vx)  "<Vx>"
  MATLAB Function1/1(g) -> Product/1
  Transfer Fcn/1 -> Product1/2
  Transfer Fcn2/1 -> Transfer Fcn/1

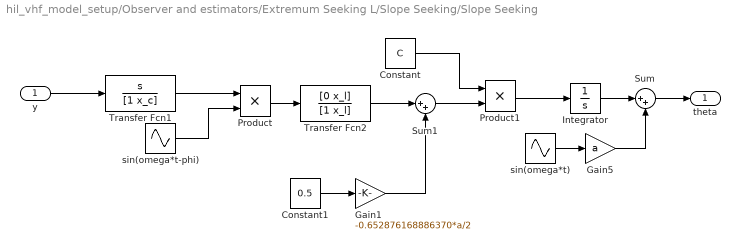
== system hil_vhf_model_setup/Observer and estimators/Extremum Seeking L/Slope Seeking/Slope Seeking ==
  y : Inport
  Constant : Constant  Value=C
  Constant1 : Constant  Value=0.5
  Gain1 : Gain  Gain=-0.652876168886370*a/2
  Gain5 : Gain  Gain=a
  Integrator : Integrator  InitialCondition=0.03  LimitOutput=on  UpperSaturationLimit=0.2  LowerSaturationLimit=0
  Product : Product
  Product1 : Product
  Sum : Sum  Inputs=|++
  Sum1 : Sum  Inputs=|++
  Transfer Fcn1 : TransferFcn  Numerator=[1 0]  Denominator=[1 x_c]
  Transfer Fcn2 : TransferFcn  Numerator=[0 x_l]  Denominator=[1 x_l]
  sin(omega*t) : Sin  Frequency=omega  SampleTime=0
  sin(omega*t-phi) : Sin  Frequency=omega  Phase=phi  SampleTime=0
  theta : Outport
  wires:
  Transfer Fcn1/1 -> Product/1
  sin(omega*t)/1 -> Gain5/1
  Gain5/1 -> Sum/2
  Sum/1 -> theta/1
  Sum1/1 -> Product1/2
  y/1 -> Transfer Fcn1/1
  sin(omega*t-phi)/1 -> Product/2
  Product1/1 -> Integrator/1
  Integrator/1 -> Sum/1
  Constant/1 -> Product1/1
  Product/1 -> Transfer Fcn2/1
  Gain1/1 -> Sum1/2
  Constant1/1 -> Gain1/1
  Transfer Fcn2/1 -> Sum1/1

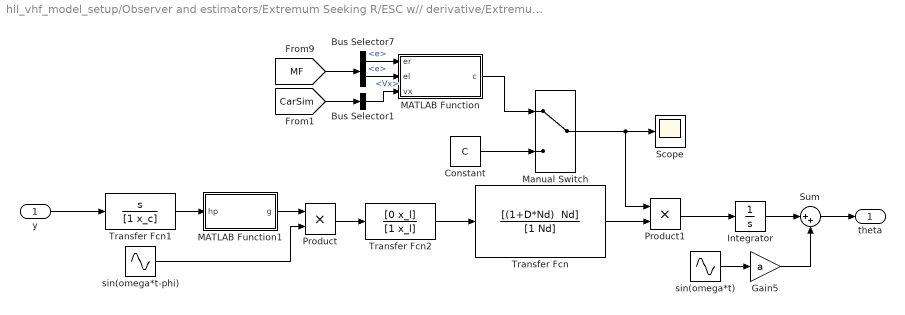
== system hil_vhf_model_setup/Observer and estimators/Extremum Seeking R/ESC w// derivative/Extremum Seeking ==
  y : Inport
  Bus Selector1 : BusSelector  OutputSignals=Vx
  Bus Selector7 : BusSelector  OutputSignals=info (signal 1).e,info (signal 2).e
  Constant : Constant  Value=C
  Gain5 : Gain  Gain=a
  Integrator : Integrator  InitialCondition=0.1  LimitOutput=on  UpperSaturationLimit=0.1  LowerSaturationLimit=0.099
  MATLAB Function : MATLAB Function  TreatAsAtomicUnit=on
  MATLAB Function1 : MATLAB Function  TreatAsAtomicUnit=on
  Manual Switch : ManualSwitch
  Product : Product
  Product1 : Product
  Scope : Scope
  Sum : Sum  Inputs=|++
  Transfer Fcn : TransferFcn  Numerator="[(1+D*Nd)  Nd]"  Denominator=[1 Nd]
  Transfer Fcn1 : TransferFcn  Numerator=[1 0]  Denominator=[1 x_c]
  Transfer Fcn2 : TransferFcn  Numerator=[0 x_l]  Denominator=[1 x_l]
  sin(omega*t) : Sin  Frequency=omega  SampleTime=0
  sin(omega*t-phi) : Sin  Frequency=omega  Phase=phi  SampleTime=0
  theta : Outport
  wires:
  sin(omega*t)/1 -> Gain5/1
  Gain5/1 -> Sum/2
  Sum/1 -> theta/1
  Product/1 -> Transfer Fcn2/1
  y/1 -> Transfer Fcn1/1
  sin(omega*t-phi)/1 -> Product/2
  Product1/1 -> Integrator/1
  Integrator/1 -> Sum/1
  [MF] -> Bus Selector7/1
  Bus Selector7/1 -> MATLAB Function/1(er)  "<e>"
  Bus Selector7/2 -> MATLAB Function/2(el)  "<e>"
  MATLAB Function/1(c) -> Manual Switch/1
  Constant/1 -> Manual Switch/2
  Manual Switch/1 -> Product1/1, Scope/1
  Transfer Fcn1/1 -> MATLAB Function1/1(hp)
  [CarSim] -> Bus Selector1/1
  Bus Selector1/1 -> MATLAB Function/3(vx)  "<Vx>"
  MATLAB Function1/1(g) -> Product/1
  Transfer Fcn/1 -> Product1/2
  Transfer Fcn2/1 -> Transfer Fcn/1

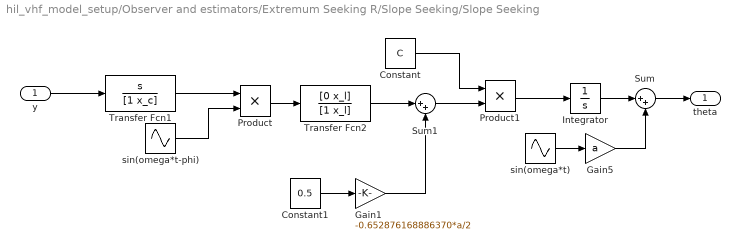
== system hil_vhf_model_setup/Observer and estimators/Extremum Seeking R/Slope Seeking/Slope Seeking ==
  y : Inport
  Constant : Constant  Value=C
  Constant1 : Constant  Value=0.5
  Gain1 : Gain  Gain=-0.652876168886370*a/2
  Gain5 : Gain  Gain=a
  Integrator : Integrator  InitialCondition=0.03  LimitOutput=on  UpperSaturationLimit=0.2  LowerSaturationLimit=0
  Product : Product
  Product1 : Product
  Sum : Sum  Inputs=|++
  Sum1 : Sum  Inputs=|++
  Transfer Fcn1 : TransferFcn  Numerator=[1 0]  Denominator=[1 x_c]
  Transfer Fcn2 : TransferFcn  Numerator=[0 x_l]  Denominator=[1 x_l]
  sin(omega*t) : Sin  Frequency=omega  SampleTime=0
  sin(omega*t-phi) : Sin  Frequency=omega  Phase=phi  SampleTime=0
  theta : Outport
  wires:
  Transfer Fcn1/1 -> Product/1
  sin(omega*t)/1 -> Gain5/1
  Gain5/1 -> Sum/2
  Sum/1 -> theta/1
  Sum1/1 -> Product1/2
  y/1 -> Transfer Fcn1/1
  sin(omega*t-phi)/1 -> Product/2
  Product1/1 -> Integrator/1
  Integrator/1 -> Sum/1
  Constant/1 -> Product1/1
  Product/1 -> Transfer Fcn2/1
  Gain1/1 -> Sum1/2
  Constant1/1 -> Gain1/1
  Transfer Fcn2/1 -> Sum1/1

== matlab function hil_vhf_model_setup/Observer and estimators/Extremum Seeking L/ESC w// derivative/Extremum Seeking/MATLAB Function ==
  data: er input; c output; el input; C parameter; vx input
function c = fcn(er, el, C, vx)

persistent de_ant;
persistent e_ant;
if(isempty(de_ant)||isempty(e_ant))
    de_ant = 0;
    e_ant = 0;
end

e = (er+el)/2;

if(e^2<1e-4)
    c = C;
else
    c = C*(exp(-(e^2)/0.0001));
end
% c=C;
if(vx>80 || vx<0.1)
    c=0;
end
% de = 19.03*(e-e_ant)+0.9048*de_ant;
% 
% if(abs(e)>0.01 || abs(de)>0.05)
%     c=0;
% else
%     c = C;
% end

% if(j<=0)
%     y = 0;
% else
%     y = 200*j;
% end

== matlab function hil_vhf_model_setup/Observer and estimators/MATLAB Function ==
  data: u input; y input; xhat output; Lc parameter
function xhat  = kalmanFilter(u, y, Lc)

persistent xhat_ant;    % last state
persistent y_ant;       % last output
persistent u_ant;       % last input
persistent P;
persistent R;
persistent Q;
persistent n;           % state vector size
persistent k;           % input vector size
persistent r;           % output vector size


A = [1,-2.890291064522695e-04;0,1];
B = [0.001;0];
C = [1, 0];
D = 0;
Psi = [-0.289029106452270,0;0,2];

if(isempty(xhat_ant)||isempty(y_ant)||isempty(u_ant)||isempty(n)||isempty(k)||isempty(r)||isempty(P)||isempty(Q)||isempty(R))
    n = size(A,1);
    k = size(u,1);
    r = size(y,1);
    xhat_ant = zeros(n,1);
    y_ant = zeros(r,1);
    u_ant = zeros(k,1);
    
    P = zeros(n);
    R = 0;
    Q = diag([0 100]);
end

%current_mea_estimator = true;
% Prediction
xbar = A*xhat_ant + B*u;
% Correction
xhat = xbar + Lc*(y-C*xbar);

% % Prediction
% xbar = A*xhat_ant + B*u;
% M = A*P*A.' + 
% % Correction
% xhat = xbar + Lc*(y-C*xbar);

xhat_ant = xhat;
u_ant = u;
y_ant = y;

== matlab function hil_vhf_model_setup/Observer and estimators/Extremum Seeking L/ESC w// derivative/Extremum Seeking/MATLAB Function1 ==
  data: hp input; g output
function g = demAmp(hp)

% if(abs(hp)>0.05)
%     g = hp*(exp(-(abs(hp)-0.05)/0.01));
% else
%     g = hp;
% end

% g = hp*(exp(-hp^2/0.005));
g = hp;

== matlab function hil_vhf_model_setup/Observer and estimators/Extremum Seeking R/ESC w// derivative/Extremum Seeking/MATLAB Function ==
  data: er input; c output; el input; C parameter; vx input
function c = fcn(er, el, C, vx)

persistent de_ant;
persistent e_ant;
if(isempty(de_ant)||isempty(e_ant))
    de_ant = 0;
    e_ant = 0;
end

e = (er+el)/2;

if(e^2<1e-4)
    c = C;
else
    c = C*(exp(-(e^2)/0.0001));
end
% c=C;
if(vx>80 || vx<0.1)
    c=0;
end
% de = 19.03*(e-e_ant)+0.9048*de_ant;
% 
% if(abs(e)>0.01 || abs(de)>0.05)
%     c=0;
% else
%     c = C;
% end

% if(j<=0)
%     y = 0;
% else
%     y = 200*j;
% end

== matlab function hil_vhf_model_setup/Observer and estimators/Extremum Seeking R/ESC w// derivative/Extremum Seeking/MATLAB Function1 ==
  data: hp input; g output
function g = demAmp(hp)

% if(abs(hp)>0.05)
%     g = hp*(exp(-(abs(hp)-0.05)/0.01));
% else
%     g = hp;
% end

% g = hp*(exp(-hp^2/0.005));
g = hp;

== matlab function hil_vhf_model_setup/Observer and estimators/MATLAB Function1 ==
  settings: updateMethod=DISCRETE  sampleTime=0.001
  data: AVy input; slip output; mu input; dmu_ds output
function [slip,dmu_ds] = fcn(AVy, mu)

persistent mu_ant;
persistent slip_L_ant;
persistent slip_R_ant;

if(isempty(mu_ant)||isempty(slip_L_ant)||isempty(slip_R_ant))
    mu_ant = [0; 0];
    slip_L_ant = 0;
    slip_R_ant = 0;
end

slip_L = (AVy(3)-AVy(1))/max([AVy(1) 2/3.6/0.284]);
slip_R = (AVy(4)-AVy(2))/max([AVy(2) 2/3.6/0.284]);
slip = [slip_L; slip_R];

dmu_ds = [(mu(1) - mu_ant(1))/max([(slip_L - slip_L_ant) 0.00001]);...
           (mu(2) - mu_ant(2))/max([(slip_R - slip_R_ant) 0.00001])];

mu_ant = mu;
slip_L_ant = slip_L;
slip_R_ant = slip_R;
